simulink model "simulate_bandwidth_controller"  (R2026a)
settings: Solver=VariableStepAuto
settings Model: Creator=Ankit  LastModifiedBy=Ankit

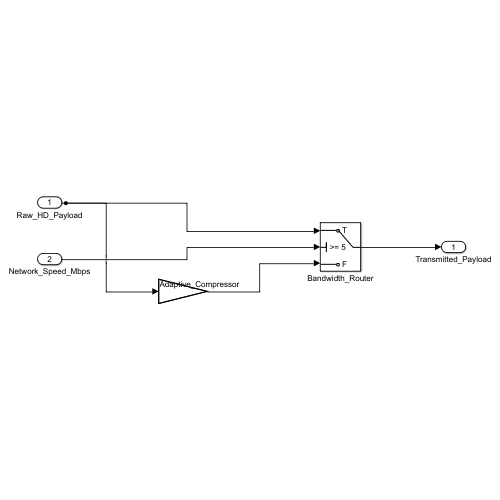
[thumbnail: Simulink's stored preview of the top-level diagram]
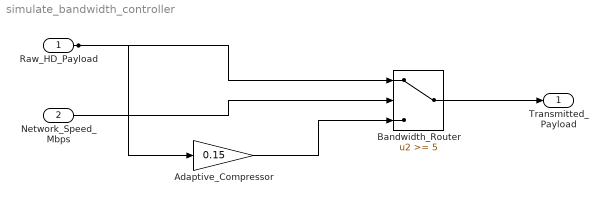
== system simulate_bandwidth_controller ==
  Raw_HD_Payload : Inport
  Network_Speed_Mbps : Inport  Port=2
  Adaptive_Compressor : Gain  Gain=0.15
  Bandwidth_Router : Switch  Threshold=5  SaturateOnIntegerOverflow=off  InputSameDT=off
  Transmitted_Payload : Outport
  wires:
  Raw_HD_Payload/1 -> Bandwidth_Router/1, Adaptive_Compressor/1
  Network_Speed_Mbps/1 -> Bandwidth_Router/2
  Adaptive_Compressor/1 -> Bandwidth_Router/3
  Bandwidth_Router/1 -> Transmitted_Payload/1
